simulink model "System1"  (R2013b)
settings: Solver=ode45  StartTime=0.0  StopTime=86400  RelTol=1e-3
libraries: cstblocks x2, simulink x1
settings Model: Creator=Patrick Robichaud  LastModifiedBy=Patrick Robichaud

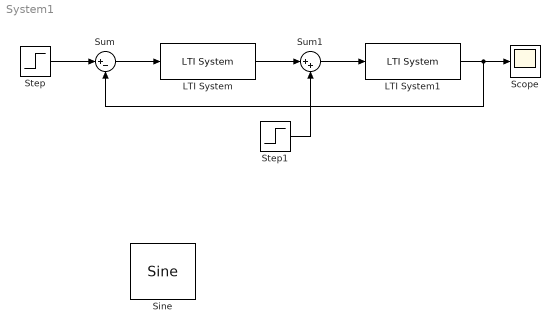
== system System1 ==
  LTI System : cstblocks/LTI System  sys=K1  IC=[]
  LTI System1 : cstblocks/LTI System  sys=G  IC=[]
  Scope : Scope
      settings: TimeRange=100  YMin=0  YMax=35
  Sine : simulink/Lookup Tables/Sine  Formula=sin(2*pi*u)  NumDataPoints=(2^5)+1  OutputWordLength=16  InternalRulePriority=Speed
  Step : Step  After=10  SampleTime=0
  Step1 : Step  After=0  SampleTime=0
  Sum : Sum  Inputs=|+-
  Sum1 : Sum  Inputs=|++
  wires:
  Sum/1 -> LTI System/1
  LTI System/1 -> Sum1/1
  Step/1 -> Sum/1
  Sum1/1 -> LTI System1/1
  LTI System1/1 -> Sum/2, Scope/1
  Step1/1 -> Sum1/2
